simulink model "Buck_Converter"  (R2021b)
settings: Solver=VariableStepAuto  StartTime=0.0  StopTime=0.05  RelTol=1e-3
libraries: spsSeriesRLCBranchLib x3, spsDCVoltageSourceLib x2, spsCurrentMeasurementLib x1, spsDiodeLib x1, spsMosfetLib x1, spsPWMGeneratorDCDCLib x1, spsVoltageMeasurementLib x1, spspowerguiLib x1
settings Model: Creator=Emre Çakmakyurdu  LastModifiedBy=Emre Çakmakyurdu

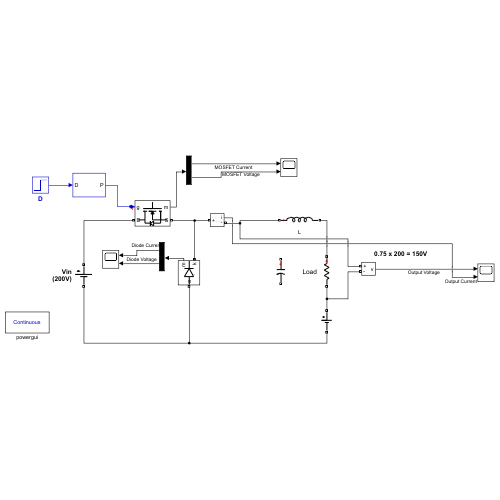
[thumbnail: Simulink's stored preview of the top-level diagram]
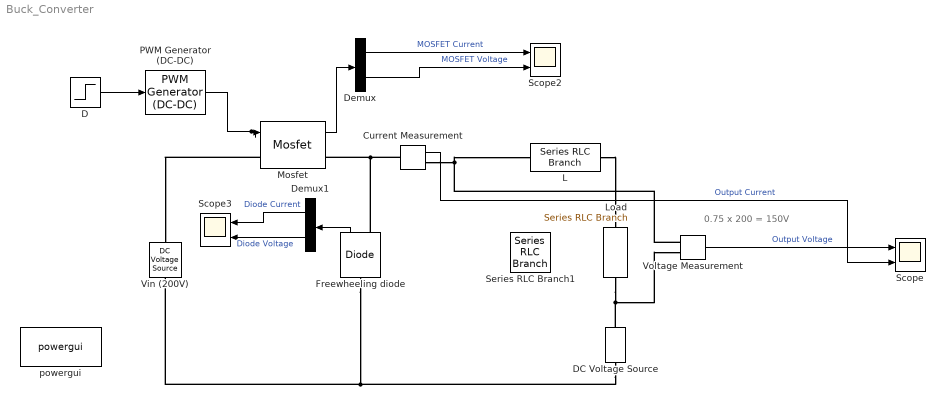
== system Buck_Converter ==
  note: 0.75 x 200 = 150V
  Current Measurement : spsCurrentMeasurementLib/Current Measurement  PhasorSimulation=off  OutputType=Complex  PSBequivalent=0
  D : Step  Time=0  Before=0.1  After=0.1  SampleTime=0
  DC Voltage Source : spsDCVoltageSourceLib/DC Voltage Source  Amplitude=0.1  Measurements=None
  Demux : Demux  Outputs=2
  Demux1 : Demux  Outputs=2
  Freewheeling diode : spsDiodeLib/Diode  Ron=0  Lon=0  Vf=0  IC=0  UseSnubber=off  Rs=inf  Cs=0  Measurements=on
  L : spsSeriesRLCBranchLib/Series RLC Branch  LConnTagsString=__new0  RConnTagsString=__new0  BranchType=L  Resistance=0.02  Inductance=24e-3  SetiL0=off  InitialCurrent=0  Capacitance=1e-6  Setx0=off  InitialVoltage=0  Measurements=None
  Load : spsSeriesRLCBranchLib/Series RLC Branch  LConnTagsString=__new0  RConnTagsString=__new0  BranchType=R  Resistance=1.07  Inductance=200e-6  SetiL0=off  InitialCurrent=0  Capacitance=400e-6  Setx0=off  InitialVoltage=0  Measurements=None
  Mosfet : spsMosfetLib/Mosfet  Ron=0.1  Lon=0  Rd=0.01  Vfd=0  IC=0  Rs=1e5  Cs=inf  Measurements=on
  PWM Generator (DC-DC) : spsPWMGeneratorDCDCLib/PWM Generator (DC-DC)  Fsw=1e3  Ts=0
  Scope : Scope  NumInputPorts=2
  Scope2 : Scope  NumInputPorts=2
  Scope3 : Scope  NumInputPorts=2
  Series RLC Branch1 : spsSeriesRLCBranchLib/Series RLC Branch  LConnTagsString=__new0  RConnTagsString=__new0  BranchType=C  Resistance=1e-4  Inductance=200e-6  SetiL0=off  InitialCurrent=0  Capacitance=30e-6  Setx0=off  InitialVoltage=150  Measurements=None
  Vin (200V) : spsDCVoltageSourceLib/DC Voltage Source  Amplitude=200  Measurements=None
  Voltage Measurement : spsVoltageMeasurementLib/Voltage Measurement  PhasorSimulation=off  OutputType=Complex  PSBequivalent=0
  powergui : spspowerguiLib/powergui  Priority=1  SimulationMode=Continuous  SampleTime=50e-6  frequency=60  Iterations=50  frequencyindice=0  Pbase=100e6  ErrMax=1e-4  UnitsV=kV  UnitsW=MW  buscounter=0  FunctionMessages=off  echomessages=off  EnableUseOfTLC=off  CurrentSourceSwitches=off  DisableSnubberDevices=off  DisableRonSwitches=off  DisableVfSwitches=off  DisplayEquations=off  AutomaticDiscreteSolvers=off  SolverType=Tustin/Backward Euler (TBE)  Interpol=off  ExternalGateDelay=off  methode=off  Ts=100  x0status=blocks  SPID=on  SwTol=0  HookPort=off  NonlinearTolerance=1e-4  nMaxIteration=100  ContinueOnMaxIteration=off  RestoreLinks=warning  ResistiveCurrentMeasurement=off  Frange=[0:2:500]  Ylog=off  Xlog=on  ShowGrid=off  save=off  variable=ZData  structure=0  ZoomFFT=off  StartTime=0.0  cycles=1  DisplayStyle=1  fundamental=60  FreqAxis=off  MaxFrequency=1000  frequencyindicesteady=1  RmsSteady=1  display=off
  wires:
  Voltage Measurement/1 -> Scope/1  "Output Voltage"
  D/1 -> PWM Generator (DC-DC)/1
  PWM Generator (DC-DC)/1 -> Mosfet/1
  Demux/1 -> Scope2/1  "MOSFET Current"
  Demux/2 -> Scope2/2  "MOSFET Voltage"
  Mosfet/1 -> Demux/1
  Freewheeling diode/1 -> Demux1/1
  Demux1/2 -> Scope3/2  "Diode Voltage"
  Demux1/1 -> Scope3/1  "Diode Current"
  Current Measurement/1 -> Scope/2  "Output Current"
  connections:
  L/RConn1 -- Load/LConn1
  Freewheeling diode/LConn1 -- DC Voltage Source/LConn1 -- Vin (200V)/LConn1
  Freewheeling diode/RConn1 -- Current Measurement/LConn1 -- Mosfet/RConn1
  Load/RConn1 -- DC Voltage Source/RConn1 -- Voltage Measurement/LConn2
  Mosfet/LConn1 -- Vin (200V)/RConn1
  Voltage Measurement/LConn1 -- L/LConn1 -- Current Measurement/RConn1
